simulink model "inverted_pendulum"  (R2012b)
settings: Solver=ode45  StartTime=0.0  StopTime=10.0  RelTol=1e-3
values from neighbouring files (symbols this model uses):
  g = 9.8    [constants.m]
  L = 0.5    [constants.m]
  m = 0.1    [constants.m]
  m_c = 1    [constants.m]
settings Model: Creator=vsnikkil  LastModifiedBy=vesa
settings OptimizationCC: InlineParams=on

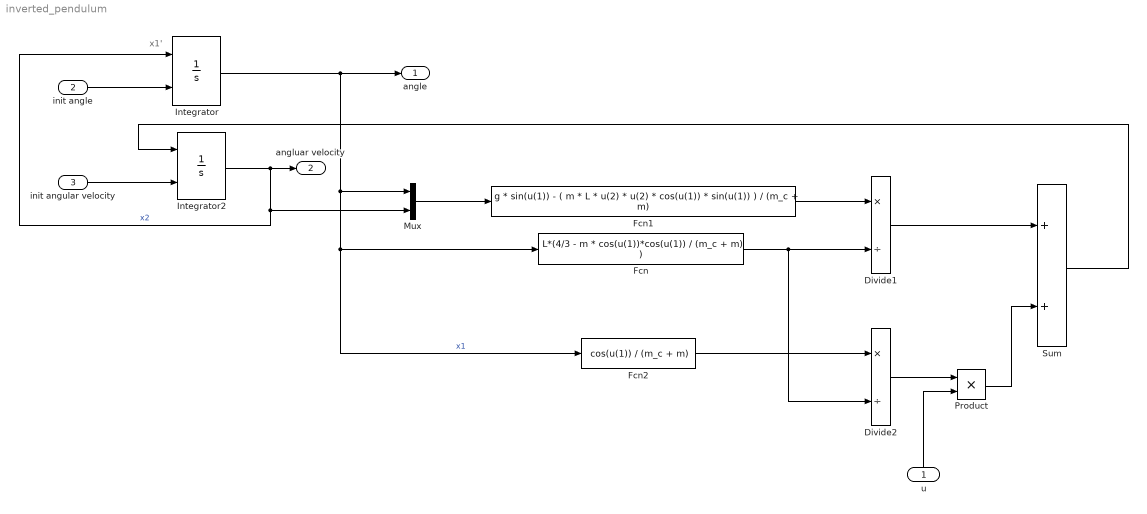
== system inverted_pendulum ==
  note: x1'
  u : Inport
  init angle : Inport  Port=2
  init angular velocity : Inport  Port=3
  Divide1 : Product  Inputs=*/
  Divide2 : Product  Inputs=*/
  Fcn : Fcn  Expr="L*(4/3 - m * cos(u(1))*cos(u(1)) / (m_c + m)   )"
  Fcn1 : Fcn  Expr=g * sin(u(1)) - ( m * L * u(2) * u(2) * cos(u(1)) * sin(u(1)) ) / (m_c + m)
  Fcn2 : Fcn  Expr=cos(u(1)) / (m_c + m)
  Integrator : Integrator  InitialConditionSource=external  LimitOutput=on  UpperSaturationLimit=pi/2  LowerSaturationLimit=-pi/2
  Integrator2 : Integrator  InitialConditionSource=external
  Mux : Mux  Inputs=2
  Product : Product  RndMeth=Zero
  Sum : Sum
  angle : Outport
  angluar velocity : Outport  Port=2
  wires:
  Integrator2/1 -> Mux/2, Integrator/1, angluar velocity/1  "x2"
  Integrator/1 -> angle/1, Fcn/1, Fcn2/1, Mux/1  "x1"
  Fcn1/1 -> Divide1/1
  Fcn/1 -> Divide2/2, Divide1/2
  Fcn2/1 -> Divide2/1
  Mux/1 -> Fcn1/1
  Divide1/1 -> Sum/1
  Product/1 -> Sum/2
  Divide2/1 -> Product/1
  u/1 -> Product/2
  Sum/1 -> Integrator2/1
  init angle/1 -> Integrator/2
  init angular velocity/1 -> Integrator2/2
